simulink model "pidd2"  (R2024b)
settings: Solver=VariableStepAuto  StartTime=0.0  StopTime=10.0  RelTol=1e-3
settings Model: Creator=Pramod C  LastModifiedBy=Pramod C

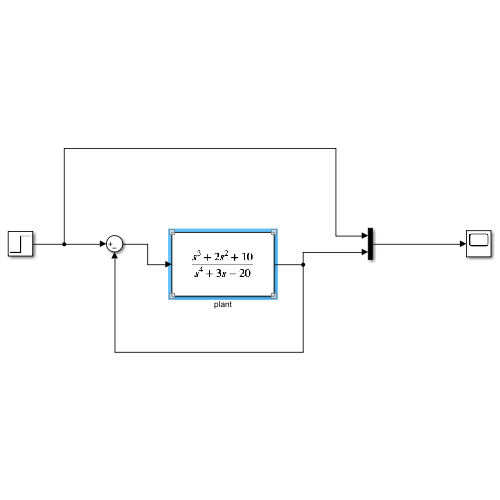
[thumbnail: Simulink's stored preview of the top-level diagram]
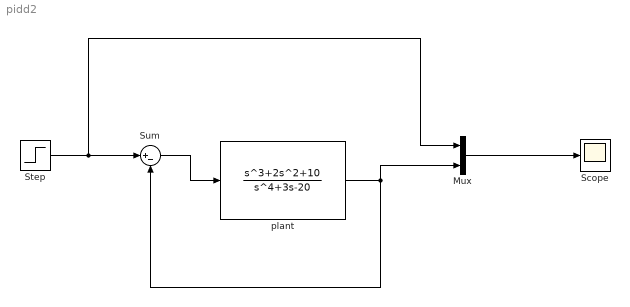
== system pidd2 ==
  Mux : Mux  Inputs=2
  Scope : Scope
  Step : Step  SampleTime=0
  Sum : Sum  Inputs=|+-
  plant : TransferFcn  Numerator=[1 2 0 10]  Denominator=[1 0 0 3 -20]
  wires:
  Sum/1 -> plant/1
  Mux/1 -> Scope/1
  Step/1 -> Mux/1, Sum/1
  plant/1 -> Mux/2, Sum/2
